simulink model "nonlinearModel"  (R2019a)
settings: Solver=ode45  StartTime=0.0  StopTime=SimulationTime  MaxStep=maxstep  RelTol=rtol
undefined symbols (not defined in the file or in its folder): beta_operating, C_Alpha, C_DX, C_DY, C_M, ePhi, F_T, g, I_CoM, initialCondition, L, m
libraries: simulink x1, dspsigops x1
settings Model: Creator=000  LastModifiedBy=000

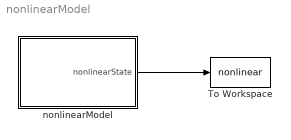
== system nonlinearModel ==
  To Workspace : ToWorkspace  VariableName=nonlinear  SaveFormat=Timeseries  SampleTime=-1
  nonlinearModel : Subsystem
  wires:
  nonlinearModel/1("nonlinearState ") -> To Workspace/1

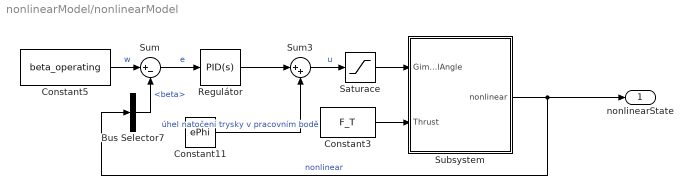
== system nonlinearModel/nonlinearModel ==
  Bus Selector7 : BusSelector  OutputSignals=beta
  Constant11 : Constant  Value=ePhi
  Constant3 : Constant  Value=F_T
  Constant5 : Constant  Value=beta_operating
  Regulátor : simulink/Continuous/PID Controller  Controller=PID  Form=Parallel  TimeDomain=Continuous-time  SampleTime=-1  IntegratorMethod=Forward Euler  FilterMethod=Forward Euler  ControllerParametersSource=internal  P=-4.14526530426782  I=-0.338776014838026  D=1.82151949632533  UseFilter=on  N=1.42272875210404  TunerSelectOption=Transfer Function Based (PID Tuner App)  InitialConditionSource=internal  InitialConditionForIntegrator=0  InitialConditionForFilter=0  DifferentiatorICPrevScaledInput=0  ExternalReset=none  TrackingMode=off  Kt=1  LimitOutput=on  UpperSaturationLimit=pi/4-ePhi  LowerSaturationLimit=-pi/4-ePhi  LinearizeAsGain=on  AntiWindupMode=back-calculation  Kb=1  POutMin=[]  POutMax=[]  IOutMin=[]  IOutMax=[]  DOutMin=[]  DOutMax=[]  NOutMin=[]  NOutMax=[]  SumOutMin=[]  SumOutMax=[]  SaturationOutMin=[]  SaturationOutMax=[]  PParamMin=[]  PParamMax=[]  IParamMin=[]  IParamMax=[]  DParamMin=[]  DParamMax=[]  NParamMin=[]  NParamMax=[]  KbParamMin=[]  KbParamMax=[]  KtParamMin=[]  KtParamMax=[]  KbOutMin=[]  KbOutMax=[]  KtOutMin=[]  KtOutMax=[]  IntegratorOutMin=[]  IntegratorOutMax=[]  FilterOutMin=[]  FilterOutMax=[]  SumI1OutMin=[]  SumI1OutMax=[]  SumI2OutMin=[]  SumI2OutMax=[]  SumI3OutMin=[]  SumI3OutMax=[]  SumI4OutMin=[]  SumI4OutMax=[]  SumDOutMin=[]  SumDOutMax=[]  DifferentiatorOutMin=[]  DifferentiatorOutMax=[]  FilterDiffOutCoefMin=[]  FilterDiffOutCoefMax=[]  ReciprocalOutMin=[]  ReciprocalOutMax=[]  SumDenOutMin=[]  SumDenOutMax=[]  SumNumOutMin=[]  SumNumOutMax=[]  DivideOutMin=[]  DivideOutMax=[]  IntegratorContinuousStateAttributes=''  IntegratorStateMustResolveToSignalObject=off  IntegratorRTWStateStorageClass=Auto  FilterContinuousStateAttributes=''  FilterStateMustResolveToSignalObject=off  FilterRTWStateStorageClass=Auto  ParallelPVariant=InternalParameters  IdealPVariant=Disabled  IVariant=InternalParameters  DVariant=InternalParameters  IntegratorVariant=Continuous  SatVariant=Enabled  AWVariant=BackCalculation  PCopyVariant=Disabled  TRVariant=Disabled  FdbkBlocksVariant=Forward  IdealPFdbkVariant=Disabled  SatFdbkVariant=Disabled  DerivativeFilterVariant=ContFilter  NVariant=InternalParameters  NCopyVariant=Disabled  FilterICVariant=InternalICsFilter  IntegratorICVariant=InternalICs  ExternalResetVariant=Disabled  TRSumVariant=Passthrough  SumFdbkVariant=Disabled  SumVariant=Sum_PID
  Saturace : Saturate  UpperLimit=pi/4  LowerLimit=-pi/4
  Subsystem : Subsystem
  Sum : Sum  Inputs=|+-
  Sum3 : Sum  Inputs=|++
  "nonlinearState " : Outport
  wires:
  Constant11/1 -> Sum3/2  "úhel natočení trysky v pracovním bodě"
  Saturace/1 -> Subsystem/1("GimbalAngle ")
  Bus Selector7/1 -> Sum/2  "<beta>"
  Sum/1 -> Regulátor/1  "e"
  Sum3/1 -> Saturace/1  "u"
  Subsystem/1(nonlinear) -> "nonlinearState "/1, Bus Selector7/1  "nonlinear"
  Constant5/1 -> Sum/1  "w"
  Regulátor/1 -> Sum3/1
  Constant3/1 -> Subsystem/2("Thrust ")

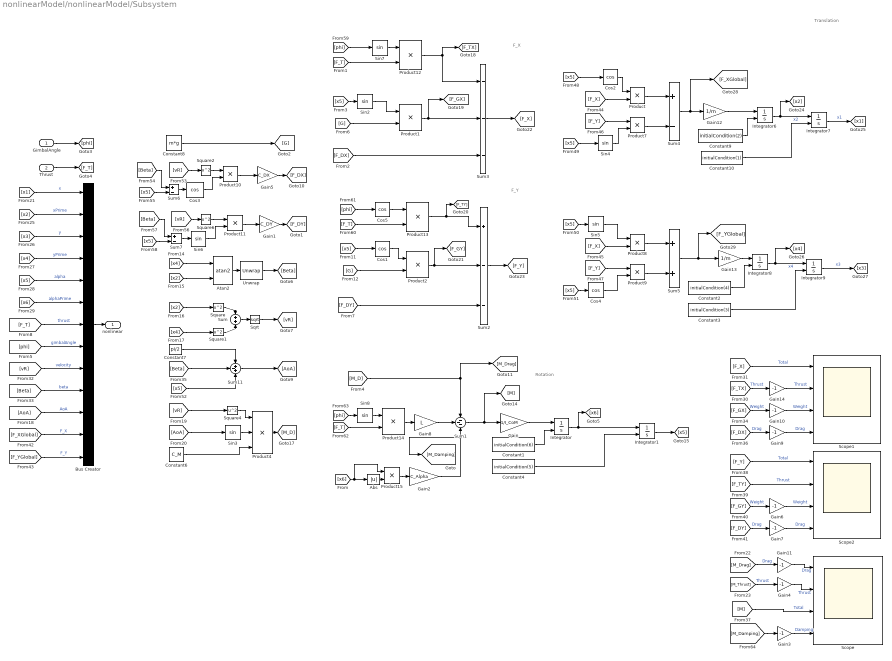
== system nonlinearModel/nonlinearModel/Subsystem ==
  note: Rotation
  note: F_X
  note: F_Y
  note: Translation
  "GimbalAngle " : Inport
  "Thrust " : Inport  Port=2
  Abs : Abs
  Atan2 : Trigonometry  Operator=atan2
  Bus Creator : BusCreator  Inputs=13
  Constant1 : Constant  Value=initialCondition(6)
  Constant10 : Constant  Value=initialCondition(1)
  Constant2 : Constant  Value=initialCondition(4)
  Constant3 : Constant  Value=initialCondition(3)
  Constant4 : Constant  Value=initialCondition(5)
  Constant6 : Constant  Value=C_M
  Constant7 : Constant  Value=pi/2
  Constant8 : Constant  Value=m*g
  Constant9 : Constant  Value=initialCondition(2)
  Cos{1..5} (5 alike) : Trigonometry  Operator=cos
  Gain : Gain  Gain=1/I_CoM
  Gain1 : Gain  Gain=C_DY
  Gain{3..4,6..7,9..11,14} (8 alike) : Gain  Gain=-1
  Gain12 : Gain  Gain=1/m
  Gain13 : Gain  Gain=1/m
  Gain2 : Gain  Gain=C_Alpha
  Gain5 : Gain  Gain=C_DX
  Gain8 : Gain  Gain=L
  Integrator{,1,6..9} (6 alike) : Integrator  InitialConditionSource=external
  Product{,1..2,7..15} (12 alike) : Product
  Product4 : Product  Inputs=3
  Scope : Scope  NumInputPorts=4
  Scope1 : Scope  NumInputPorts=4
  Scope2 : Scope  NumInputPorts=4
  Sin{2..8} (7 alike) : Trigonometry
  Sqrt : Sqrt  SaturateOnIntegerOverflow=on
  Square{,1..2,4,6} (5 alike) : Math  Operator=square  SaturateOnIntegerOverflow=on
  Sum : Sum
  Sum1 : Sum  Inputs=---
  Sum11 : Sum  Inputs=+-+
  Sum2 : Sum  Inputs=+--
  Sum3 : Sum  Inputs=---
  Sum4 : Sum  Inputs=+-
  Sum5 : Sum
  Sum6 : Sum  Inputs=+-
  Sum7 : Sum  Inputs=+-
  Unwrap : dspsigops/Unwrap  tol=pi  running=off
  nonlinear : Outport
  wires:
  Integrator1/1 -> [x5]
  Sum1/1 -> [M], Gain/1
  Sum2/1 -> [F_Y]
  [x6] -> Bus Creator/6  "alphaPrime"
  [Beta] -> Sum11/2
  Sum3/1 -> [F_X]
  Constant1/1 -> Integrator/2
  Square1/1 -> Sum/2
  [x5] -> Bus Creator/5  "alpha"
  [x2] -> Bus Creator/2  "xPrime"
  Square/1 -> Sum/1
  Sum/1 -> Sqrt/1
  Integrator/1 -> [x6], Integrator1/1
  [x4] -> Bus Creator/4  "yPrime"
  Gain/1 -> Integrator/1
  [x3] -> Bus Creator/3  "y"
  Constant4/1 -> Integrator1/2
  Sqrt/1 -> [vR]
  Atan2/1 -> Unwrap/1
  [x1] -> Bus Creator/1  "x"
  [M_Drag] -> Gain11/1  "Drag"
  Constant7/1 -> Sum11/1
  Unwrap/1 -> [Beta]
  Sum11/1 -> [AoA]
  [M] -> Scope/3  "Total"
  Constant8/1 -> [G]
  Gain5/1 -> [F_DX]
  [F_DX] -> Sum3/3
  Product1/1 -> Sum3/2, [F_GX]
  [x5] -> Sin2/1
  Sin2/1 -> Product1/1
  [G] -> Product1/2
  [G] -> Product2/2
  Cos1/1 -> Product2/1
  [x5] -> Cos1/1
  Product2/1 -> [F_GY], Sum2/2
  [F_DY] -> Sum2/3
  [x4] -> Atan2/1
  [x2] -> Atan2/2
  [x2] -> Square/1
  [x4] -> Square1/1
  [vR] -> Square4/1
  Square4/1 -> Product4/1
  [AoA] -> Sin3/1
  Sin3/1 -> Product4/2
  Constant6/1 -> Product4/3
  Product4/1 -> [M_D]
  [F_X] -> Scope1/1  "Total"
  [F_TX] -> Gain14/1  "Thrust"
  [F_GX] -> Gain10/1  "Weight"
  [F_DX] -> Gain9/1  "Drag"
  [F_Y] -> Scope2/1  "Total"
  [F_TY] -> Scope2/2  "Thrust"
  [F_GY] -> Gain6/1  "Weight"
  [F_DY] -> Gain7/1  "Drag"
  [M_Thrust] -> Gain4/1  "Thrust"
  Gain4/1 -> Scope/2  "Thrust"
  Gain6/1 -> Scope2/3  "Weight"
  Gain7/1 -> Scope2/4  "Drag"
  Gain9/1 -> Scope1/4  "Drag"
  Gain10/1 -> Scope1/3  "Weight"
  [M_D] -> [M_Drag], Sum1/1
  Gain11/1 -> Scope/1  "Drag"
  Constant9/1 -> Integrator6/2
  Gain12/1 -> Integrator6/1
  Sum4/1 -> [F_XGlobal], Gain12/1
  Constant10/1 -> Integrator7/2
  Integrator6/1 -> Integrator7/1, [x2]  "x2"
  Integrator7/1 -> [x1]  "x1"
  Gain13/1 -> Integrator8/1
  Integrator9/1 -> [x3]  "x3"
  Constant2/1 -> Integrator8/2
  Integrator8/1 -> Integrator9/1, [x4]  "x4"
  Sum5/1 -> [F_YGlobal], Gain13/1
  Constant3/1 -> Integrator9/2
  [x5] -> Cos2/1
  Cos2/1 -> Product/1
  [F_X] -> Product/2
  [F_Y] -> Product7/1
  [x5] -> Sin4/1
  Sin4/1 -> Product7/2
  Product/1 -> Sum4/1
  Product7/1 -> Sum4/2
  Product9/1 -> Sum5/2
  Product8/1 -> Sum5/1
  Cos4/1 -> Product9/2
  [x5] -> Cos4/1
  [F_Y] -> Product9/1
  [F_X] -> Product8/2
  Sin5/1 -> Product8/1
  [x5] -> Sin5/1
  [x5] -> Sum11/3
  Sum6/1 -> Cos3/1
  Cos3/1 -> Product10/2
  [vR] -> Square2/1
  [Beta] -> Sum6/1
  [x5] -> Sum6/2
  Product10/1 -> Gain5/1
  Product11/1 -> Gain1/1
  [x5] -> Sum7/2
  [Beta] -> Sum7/1
  [vR] -> Square6/1
  Sin6/1 -> Product11/2
  Sum7/1 -> Sin6/1
  Gain1/1 -> [F_DY]
  [x6] -> Abs/1, Product15/1
  Gain2/1 -> Sum1/3, [M_Damping]
  "GimbalAngle "/1 -> [phi]
  "Thrust "/1 -> [F_T]
  [F_T] -> Product12/2
  Sin7/1 -> Product12/1
  [phi] -> Sin7/1
  Product12/1 -> [F_TX], Sum3/1
  Product13/1 -> Sum2/1, [F_TY]
  [phi] -> Cos5/1
  Cos5/1 -> Product13/1
  [F_T] -> Product13/2
  [F_T] -> Product14/2
  [phi] -> Sin8/1
  Sin8/1 -> Product14/1
  Gain8/1 -> Sum1/2
  Product14/1 -> Gain8/1
  Square2/1 -> Product10/1
  Square6/1 -> Product11/1
  [M_Damping] -> Gain3/1
  Product15/1 -> Gain2/1
  Abs/1 -> Product15/2
  [F_T] -> Bus Creator/7  "thrust"
  [phi] -> Bus Creator/8  "gimbalAngle"
  [vR] -> Bus Creator/9  "velocity"
  [Beta] -> Bus Creator/10  "beta"
  [AoA] -> Bus Creator/11  "AoA"
  [F_XGlobal] -> Bus Creator/12  "F_X"
  [F_YGlobal] -> Bus Creator/13  "F_Y"
  Gain3/1 -> Scope/4  "Damping"
  Bus Creator/1 -> nonlinear/1
  Gain14/1 -> Scope1/2  "Thrust"
